simulink model "PDInverseDynOS"  (R2020b)
settings: Solver=VariableStepAuto  StartTime=0.0  StopTime=5  RelTol=1e-3
values from neighbouring files (symbols this model uses):
  Kd = diag([50 70 50 1 1 1])    [params.m]
  Kp = diag([700 900 700 1 1 1])    [params.m]
libraries: robotcorelib x1, vrlib x1
settings Model: Creator=andre  LastModifiedBy=filippo

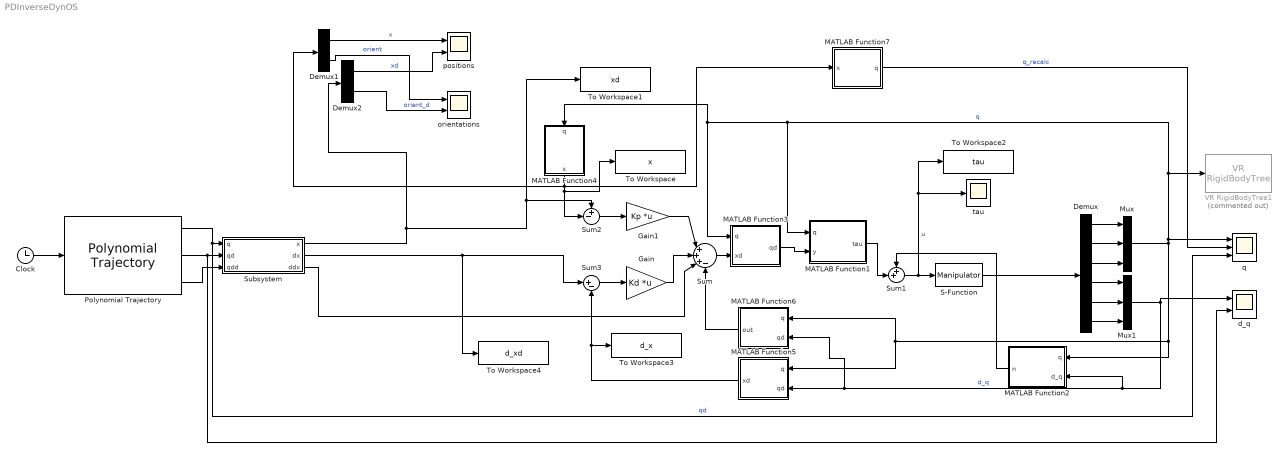
== system PDInverseDynOS ==
  Clock : Clock
  Demux : Demux  Outputs=6
  Demux1 : Demux  Outputs=2
  Demux2 : Demux  Outputs=2
  Gain : Gain  Gain=Kd  Multiplication=Matrix(K*u)
  Gain1 : Gain  Gain=Kp  Multiplication=Matrix(K*u)
  MATLAB Function1 : MATLAB Function  TreatAsAtomicUnit=on
  MATLAB Function2 : MATLAB Function  TreatAsAtomicUnit=on
  MATLAB Function3 : MATLAB Function  TreatAsAtomicUnit=on
  MATLAB Function4 : MATLAB Function  TreatAsAtomicUnit=on
  MATLAB Function5 : MATLAB Function  TreatAsAtomicUnit=on
  MATLAB Function6 : MATLAB Function  TreatAsAtomicUnit=on
  MATLAB Function7 : MATLAB Function  TreatAsAtomicUnit=on
  Mux : Mux  Inputs=3
  Mux1 : Mux  Inputs=3
  Polynomial Trajectory : robotcorelib/Polynomial Trajectory  WaypointSource=Internal  Waypoints=[0,0,0.1;0,-0.1,0;0,0.1,0]  TimePoints=[ 0, 2, 4 ]  TimeInterval=[ 1, 4 ]  Method=Quintic Polynomial  ParameterSource=Internal  VelocityBoundaryCondition=zeros(3,3)  AccelerationBoundaryCondition=zeros(3,3 )  SimulateUsing=Interpreted execution
  S-Function : S-Function  FunctionName=Manipulator  Parameters=param  SFunctionDeploymentMode=off  EnableBusSupport=off
  Subsystem : Subsystem
  Sum : Sum  Inputs=|+++-
  Sum1 : Sum  Inputs=++|
  Sum2 : Sum  Inputs=+-|
  Sum3 : Sum  Inputs=|+-
  To Workspace : ToWorkspace  VariableName=x  SaveFormat=Timeseries  SampleTime=-1
  To Workspace1 : ToWorkspace  VariableName=xd  SaveFormat=Timeseries  SampleTime=-1
  To Workspace2 : ToWorkspace  VariableName=tau  SaveFormat=Timeseries  SampleTime=-1
  To Workspace3 : ToWorkspace  VariableName=d_x  SaveFormat=Timeseries  SampleTime=-1
  To Workspace4 : ToWorkspace  VariableName=d_xd  SaveFormat=Timeseries  SampleTime=-1
  VR RigidBodyTree1 : vrlib/VR RigidBodyTree  Commented=on  RBT=robot  useRBT=on  Ts=-1  ForceViewerOpen=on
      settings: SourceProductBaseCode=SL
  d_q : Scope  NumInputPorts=2
  orientations : Scope  NumInputPorts=2
  positions : Scope  NumInputPorts=2
  q : Scope  NumInputPorts=3
  tau : Scope
  wires:
  Gain1/1 -> Sum/1
  S-Function/1 -> Demux/1
  Demux/3 -> Mux/3
  Demux/2 -> Mux/2
  Demux/1 -> Mux/1
  Demux/4 -> Mux1/1
  Demux/5 -> Mux1/2
  Demux/6 -> Mux1/3
  Mux/1 -> VR RigidBodyTree1/1, MATLAB Function4/1(q), MATLAB Function3/1(q), MATLAB Function1/1(q), q/1, MATLAB Function6/1(q), MATLAB Function5/1(q), MATLAB Function2/1(q)  "q"
  Sum1/1 -> To Workspace2/1, tau/1, S-Function/1  "u"
  Gain/1 -> Sum/2
  Mux1/1 -> MATLAB Function6/2(qd), MATLAB Function5/2(qd), MATLAB Function2/2(d_q), d_q/1  "d_q"
  MATLAB Function2/1(n) -> Sum1/1
  MATLAB Function1/1(tau) -> Sum1/2
  Sum2/1 -> Gain1/1
  Sum3/1 -> Gain/1
  Polynomial Trajectory/1 -> Subsystem/1(q), q/3  "qd"
  Sum/1 -> MATLAB Function3/2(xd)
  MATLAB Function3/1(qd) -> MATLAB Function1/2(y)
  MATLAB Function4/1(x) -> MATLAB Function7/1(x), To Workspace/1, Sum2/2, Demux1/1
  MATLAB Function5/1(xd) -> To Workspace3/1, Sum3/2
  MATLAB Function6/1(out) -> Sum/4
  Clock/1 -> Polynomial Trajectory/1
  Subsystem/1(x) -> To Workspace1/1, Sum2/1, Demux2/1
  Subsystem/3(ddx) -> Sum/3
  Subsystem/2(dx) -> Sum3/1, To Workspace4/1
  Demux1/1 -> positions/1  "x"
  Demux2/1 -> positions/2  "xd"
  Demux1/2 -> orientations/1  "orient"
  Demux2/2 -> orientations/2  "orient_d"
  Polynomial Trajectory/2 -> d_q/2, Subsystem/2(qd)
  Polynomial Trajectory/3 -> Subsystem/3(qdd)
  MATLAB Function7/1(q) -> q/2  "q_recalc"

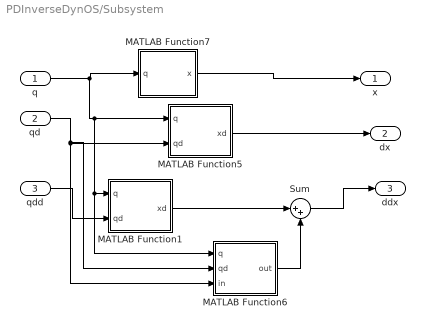
== system PDInverseDynOS/Subsystem ==
  q : Inport
  qd : Inport  Port=2
  qdd : Inport  Port=3
  MATLAB Function1 : MATLAB Function  TreatAsAtomicUnit=on
  MATLAB Function5 : MATLAB Function  TreatAsAtomicUnit=on
  MATLAB Function6 : MATLAB Function  TreatAsAtomicUnit=on
  MATLAB Function7 : MATLAB Function  TreatAsAtomicUnit=on
  Sum : Sum  Inputs=|++
  x : Outport
  dx : Outport  Port=2
  ddx : Outport  Port=3
  wires:
  q/1 -> MATLAB Function6/1(q), MATLAB Function1/1(q), MATLAB Function5/1(q), MATLAB Function7/1(q)
  MATLAB Function7/1(x) -> x/1
  MATLAB Function5/1(xd) -> dx/1
  qdd/1 -> MATLAB Function1/2(qd)
  qd/1 -> MATLAB Function6/3(in), MATLAB Function5/2(qd), MATLAB Function6/2(qd)
  MATLAB Function6/1(out) -> Sum/2
  MATLAB Function1/1(xd) -> Sum/1
  Sum/1 -> ddx/1

== matlab function PDInverseDynOS/MATLAB Function1 ==
  data: q input; y input; tau output; param parameter
function tau = B(q,y,param)
    B_matrix = B_Lagrangian(q, param);
    tau =  B_matrix * y;
end

== matlab function PDInverseDynOS/MATLAB Function3 ==
  data: q input; xd input; qd output; param parameter
function qd = invJa(q, xd, param)
    Ja = AnalyticalJacobian(q,param);
    qd = pinv(Ja) * xd;
end

== matlab function PDInverseDynOS/MATLAB Function2 ==
  data: q input; n output; d_q input; param parameter
function n = n(q,d_q,param)
    % Compute C and G used in the model of n(q,d_q)
    C = double(C_Lagrangian(q, d_q, param));
    G = double(G_Lagrangian(q, param));
    Fsv = param.Fsv;

    n = C * d_q + G + Fsv * d_q;
end

== matlab function PDInverseDynOS/MATLAB Function4 ==
  data: q input; x output; param parameter
function x = Kin(q,param)
    x = Kinematics(q,param);
end

== matlab function PDInverseDynOS/MATLAB Function5 ==
  data: q input; qd input; xd output; param parameter
function xd = Ja(q, qd, param)
    Ja = AnalyticalJacobian(q,param);
    xd = Ja * qd;
end

== matlab function PDInverseDynOS/MATLAB Function6 ==
  data: q input; qd input; out output; param parameter
function out = dot_Ja(q, qd, param)
    d_Ja = AnalyticalJacobian_dot(q,qd,param);
    out = d_Ja * qd;
end

== matlab function PDInverseDynOS/MATLAB Function7 ==
  data: x input; q output; param parameter
function q = KinInv(x,param)
    q = InverseKinematics(x,param);
end

== matlab function PDInverseDynOS/Subsystem/MATLAB Function7 ==
  data: q input; x output; param parameter
function x = Kin(q,param)
    x = Kinematics(q,param);
end

== matlab function PDInverseDynOS/Subsystem/MATLAB Function5 ==
  data: q input; qd input; xd output; param parameter
function xd = Ja(q, qd, param)
    Ja = AnalyticalJacobian(q,param);
    xd = Ja * qd;
end

== matlab function PDInverseDynOS/Subsystem/MATLAB Function1 ==
  data: q input; qd input; xd output; param parameter
function xd = Ja(q, qd, param)
    Ja = AnalyticalJacobian(q,param);
    xd = Ja * qd;
end

== matlab function PDInverseDynOS/Subsystem/MATLAB Function6 ==
  data: q input; qd input; in input; out output; param parameter
function out = dot_Ja(q, qd, in, param)
    d_Ja = AnalyticalJacobian_dot(q,qd,param);
    out = d_Ja * in;
end
